simulink model "RL"  (R2021a)
settings: Solver=VariableStepAuto  StartTime=0.0  StopTime=10.0  RelTol=1e-3
values from neighbouring files (symbols this model uses):
  L = input('L=')    [RLckt.m]    (also in motor.m = input('Enter value of L='))
  R = input('Enter value of R=')    [RC.m]    (also in RCckt.m = input('R='); RLckt.m = input('R='); motor.m)
settings Model: Creator=User  LastModifiedBy=User

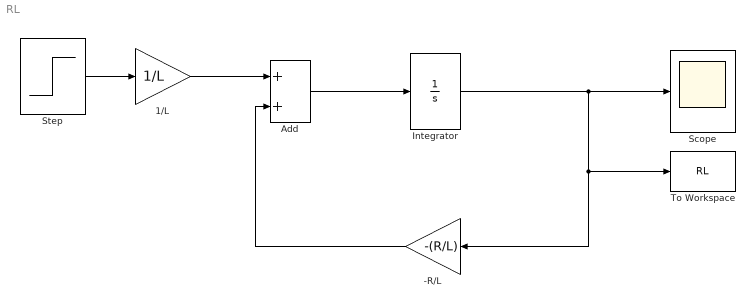
== system RL ==
  -R/L : Gain  Gain=-(R/L)
  1/L : Gain  Gain=1/L
  Add : Sum
  Integrator : Integrator
  Scope : Scope
  Step : Step  SampleTime=0
  To Workspace : ToWorkspace  VariableName=RL  SaveFormat=Timeseries  SampleTime=-1
  wires:
  Step/1 -> 1/L/1
  -R/L/1 -> Add/2
  1/L/1 -> Add/1
  Add/1 -> Integrator/1
  Integrator/1 -> To Workspace/1, -R/L/1, Scope/1
